simulink model "ver5simple"  (R2020b)
settings: Solver=ode8  StartTime=0.0  StopTime=20  FixedStep=0.00001  RelTol=1e-3
values from neighbouring files (symbols this model uses):
  c1 = 1.2801    [input_ver5.m]
  c2 = 23.99    [input_ver5.m]
  c3 = 0.52    [input_ver5.m]
  c4 = 0.03    [input_ver5.m]
  fn = m*9.81    (= 3355.02)    [input_ver5.m]
  jw = 1.13    [input_ver5.m]
  m = 342    [input_ver5.m]
  r = 0.33    [input_ver5.m]
settings Model: Creator=K E S SRINIVAS  LastModifiedBy=K E S SRINIVAS

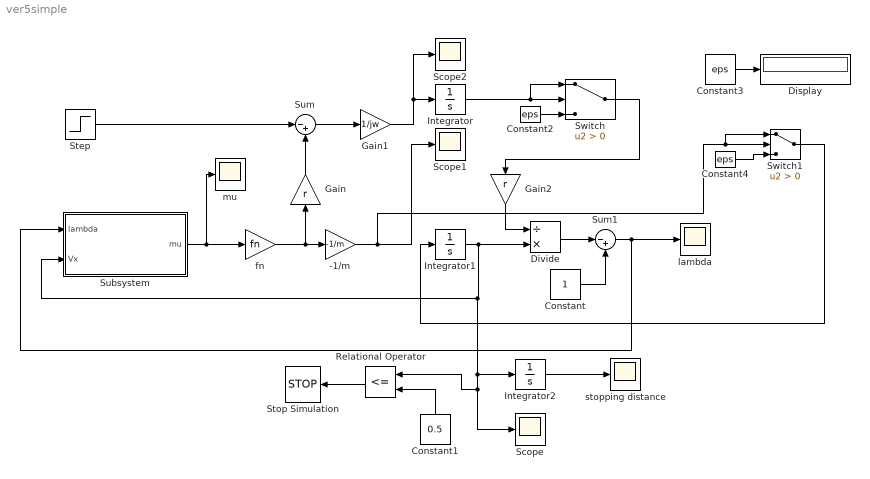
== system ver5simple ==
  -1/m : Gain  Gain=-1/m
  Constant : Constant
  Constant1 : Constant  Value=0.5
  Constant2 : Constant  Value=eps
  Constant3 : Constant  Value=eps
  Constant4 : Constant  Value=eps
  Display : Display
  Divide : Product  Inputs=/*
  Gain : Gain  Gain=r
  Gain1 : Gain  Gain=1/jw
  Gain2 : Gain  Gain=r
  Integrator : Integrator  InitialCondition=84.18  LowerSaturationLimit=0
  Integrator1 : Integrator  InitialCondition=27.78  LowerSaturationLimit=0
  Integrator2 : Integrator  LowerSaturationLimit=0
  Relational Operator : RelationalOperator  Operator=<=  OutDataTypeStr=boolean  RndMeth=Simplest
  Scope : Scope
  Scope1 : Scope
  Scope2 : Scope
  Step : Step  Time=0  After=1200  SampleTime=0
  Stop Simulation : Stop
  Subsystem : Subsystem
  Sum : Sum  Inputs=|-+
  Sum1 : Sum  Inputs=|-+
  Switch : Switch  Criteria=u2 > Threshold
  Switch1 : Switch  Criteria=u2 > Threshold
  fn : Gain  Gain=fn
  lambda : Scope
  mu : Scope
  stopping distance : Scope
  wires:
  Subsystem/1(mu) -> mu/1, fn/1
  fn/1 -> Gain/1, -1/m/1
  Step/1 -> Sum/1
  Gain/1 -> Sum/2
  Sum/1 -> Gain1/1
  Gain1/1 -> Scope2/1, Integrator/1
  Integrator1/1 -> Divide/2, Integrator2/1, Relational Operator/1, Scope/1, Subsystem/2(Vx)
  Gain2/1 -> Divide/1
  Divide/1 -> Sum1/1
  Constant/1 -> Sum1/2
  Sum1/1 -> lambda/1, Subsystem/1(lambda)
  Constant1/1 -> Relational Operator/2
  Relational Operator/1 -> Stop Simulation/1
  Integrator2/1 -> stopping distance/1
  Integrator/1 -> Switch/1, Switch/2
  Constant2/1 -> Switch/3
  Switch/1 -> Gain2/1
  Constant3/1 -> Display/1
  Switch1/1 -> Integrator1/1
  -1/m/1 -> Switch1/1, Switch1/2, Scope1/1
  Constant4/1 -> Switch1/3

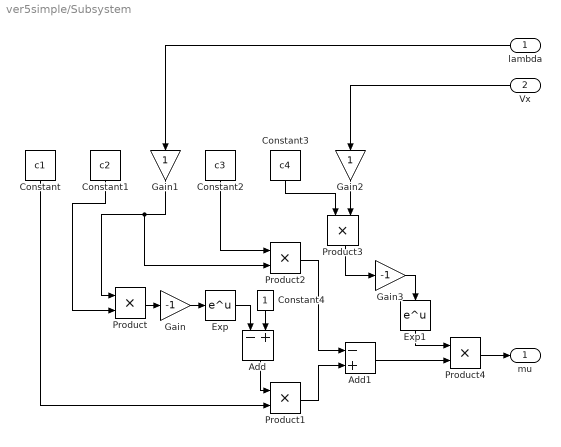
== system ver5simple/Subsystem ==
  lambda : Inport
  Vx : Inport  Port=2
  Add : Sum  Inputs=-+
  Add1 : Sum  Inputs=-+
  Constant : Constant  Value=c1
  Constant1 : Constant  Value=c2
  Constant2 : Constant  Value=c3
  Constant3 : Constant  Value=c4
  Constant4 : Constant
  Exp : Math  SaturateOnIntegerOverflow=on
  Exp1 : Math  SaturateOnIntegerOverflow=on
  Gain : Gain  Gain=-1
  Gain1 : Gain
  Gain2 : Gain
  Gain3 : Gain  Gain=-1
  Product{,1..4} (5 alike) : Product
  mu : Outport
  wires:
  Constant1/1 -> Product/2
  Gain/1 -> Exp/1
  Product1/1 -> Add1/2
  Gain3/1 -> Exp1/1
  Product/1 -> Gain/1
  Add1/1 -> Product4/2
  Gain1/1 -> Product/1, Product2/2
  Add/1 -> Product1/1
  Vx/1 -> Gain2/1
  Product3/1 -> Gain3/1
  Gain2/1 -> Product3/2
  Constant3/1 -> Product3/1
  Product4/1 -> mu/1
  Product2/1 -> Add1/1
  Exp/1 -> Add/1
  Constant2/1 -> Product2/1
  Constant4/1 -> Add/2
  Constant/1 -> Product1/2
  Exp1/1 -> Product4/1
  lambda/1 -> Gain1/1
